simulink model "Q1_Distillation_Column_Model_2x2"  (R2020b)
settings: Solver=ode45  StartTime=0.0  StopTime=450  RelTol=1e-3  EnableMultiTasking=on
settings Model: Creator=SENAI LAPTOP  LastModifiedBy=RISHIKESH_SREEKUMAR
settings DataIOCC: LimitDataPoints=on  SaveFormat=Array  ReturnWorkspaceOutputs=off
settings OptimizationCC: LifeSpan=inf
settings DebuggingCC: SolverPrmCheckMsg=warning  SFUnexpectedBacktrackingDiag=warning  SFNoUnconditionalDefaultTransitionDiag=warning  SFExecutionAtInitializationDiag=none  ArithmeticOperatorsInVariantConditions=warning
settings HardwareCC: ProdBitPerPointer=32  ProdBitPerSizeT=32  ProdBitPerPtrDiffT=32  ProdLargestAtomicFloat=None  ProdIntDivRoundTo=Undefined  ProdEndianess=Unspecified  ProdWordSize=32  ProdHWDeviceType=32-bit Generic
settings ModelReferenceCC: PropagateSignalLabelsOutOfModel=off
settings SFSimCC: SimUseLocalCustomCode=off  CustomCodeUndefinedFunction=UseInterfaceOnly
settings RTWCC: RTWUseLocalCustomCode=off
settings CodeAppCC: StateflowObjectComments=on
settings GRTTargetCC: TargetLangStandard=C89/C90 (ANSI)
settings ConfigComp: CovMetricSettings=dw  CovSaveCumulativeToWorkspaceVar=on  CovSaveSingleToWorkspaceVar=on  CovExternalEMLEnable=off  CovSFcnEnable=off

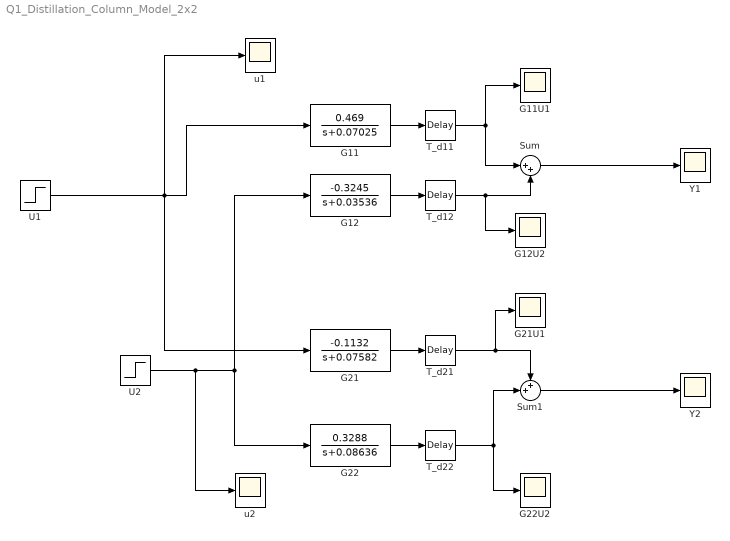
== system Q1_Distillation_Column_Model_2x2 ==
  G11 : TransferFcn  Numerator=[0.469]  Denominator=[1 0.07025]
  G11U1 : Scope
  G12 : TransferFcn  Numerator=[-0.3245]  Denominator=[1 0.03536]
  G12U2 : Scope
  G21 : TransferFcn  Numerator=[-0.1132]  Denominator=[1 0.07582]
  G21U1 : Scope
  G22 : TransferFcn  Numerator=[0.3288]  Denominator=[1 0.08636]
  G22U2 : Scope
  Sum : Sum  Inputs=|++
  Sum1 : Sum  Inputs=++|
  T_d11 : TransportDelay  DelayTime=2.5  PadeOrder=5
  T_d12 : TransportDelay  DelayTime=1.1  PadeOrder=5
  T_d21 : TransportDelay  DelayTime=1.1  PadeOrder=5
  "T_d22 " : TransportDelay  DelayTime=1.1  PadeOrder=5
  U1 : Step  Time=150  After=8  SampleTime=0.1
  U2 : Step  Time=160  After=10  SampleTime=0.1
  Y1 : Scope
  Y2 : Scope
  u1 : Scope
  u2 : Scope
  wires:
  U1/1 -> u1/1, G11/1, G21/1
  G11/1 -> T_d11/1
  Sum/1 -> Y1/1
  Sum1/1 -> Y2/1
  T_d11/1 -> G11U1/1, Sum/1
  T_d12/1 -> G12U2/1, Sum/2
  G12/1 -> T_d12/1
  T_d21/1 -> G21U1/1, Sum1/1
  G21/1 -> T_d21/1
  G22/1 -> "T_d22 "/1
  "T_d22 "/1 -> G22U2/1, Sum1/2
  U2/1 -> u2/1, G12/1, G22/1
